simulink model "primera_parte"  (R2023a)
settings: Solver=VariableStepAuto  StartTime=0.0  StopTime=3  RelTol=1e-3
values from neighbouring files (symbols this model uses):
  A = [a11 a21 a12 a22]    [calc_A.m]    (also in modelo.m = [a11 a12)
  Ad = [-1/t_beta 0 ... (first row only)    [calc_KMax.m]    (also in calc_Kmin.m; modelo.m)
  B = [b11 b21 b12 b22]    [calc_B.m]    (also in calc_inv_B.m = [b11 b12; b21 b22]; modelo.m = [b11 b12)
  C = [1 0 ... (first row only)    [modelo.m]
  D = [0 0;0 0]    [modelo.m]
  E = [e1 e2]    [calc_E.m]    (also in modelo.m = [e1)
  Ed = [k_beta/t_beta ... (first row only)    [calc_KMax.m]    (also in calc_Kmin.m; modelo.m)
  k = double(Y)*inv(double(P))    [calc_KMax.m]    (also in calc_Kmin.m; modelo.m = H_inf_robust(A1,A2,B11,B12,B21,B22,C1,D12,D11))
  x0 = [0, 0]    [modelo.m]
undefined symbols (not defined in the file or in its folder): sigbuilder_block
settings Model: Creator=Ferna  LastModifiedBy=Ferna
settings DebuggingCC: UnconnectedInputMsg=warning  UnconnectedOutputMsg=warning  UnconnectedLineMsg=warning
settings ModelReferenceCC: EnableRefExpFcnMdlSchedulingChecks=on
settings RTWCC: DLArmComputeVersion=19.05

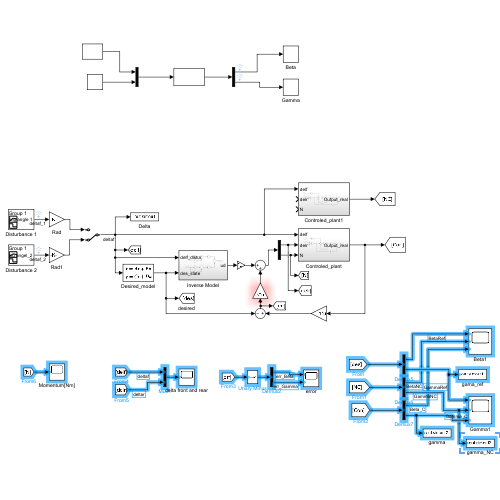
[thumbnail: Simulink's stored preview of the top-level diagram]
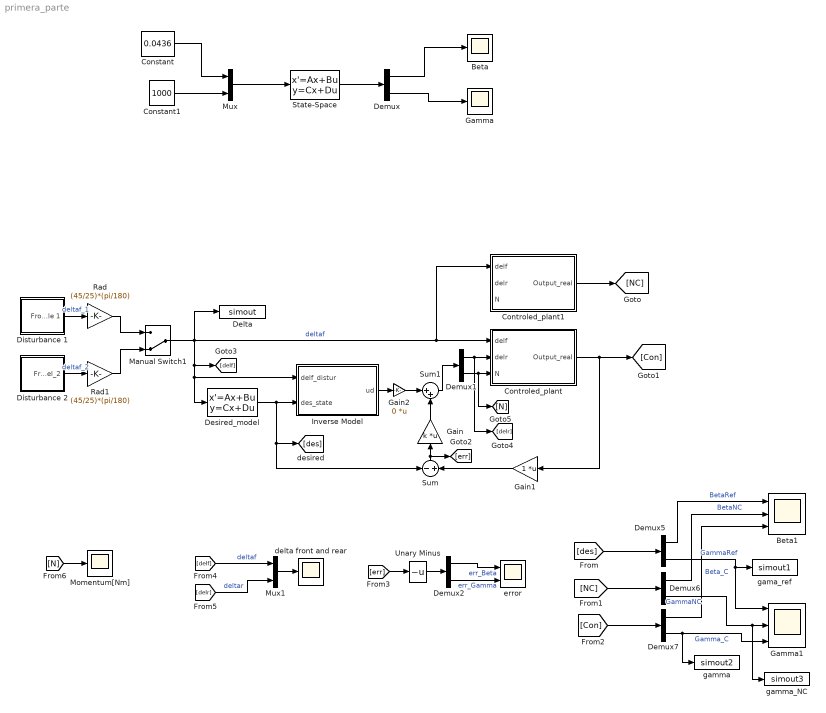
== system primera_parte ==
  Beta : Scope
  Beta1 : Scope  NumInputPorts=3
  Constant : Constant  Value=0.0436
  Constant1 : Constant  Value=1000
  Controled_plant : Subsystem
  Controled_plant1 : Subsystem
  Delta : ToWorkspace  VariableName=simout  SaveFormat=Timeseries  SampleTime=-1
  Demux{,1..2,5..7} (6 alike) : Demux  Outputs=2
  Desired_model : StateSpace  A=Ad  B=Ed  C=[1,0;0,1]  D=zeros(2,1)  InitialCondition=0
  Disturbance 1 : Subsystem  Tag=STV Subsys  LoadFcn=sigbuilder_block('load');  StartFcn=sigbuilder_block('start');  StopFcn=sigbuilder_block('stop');  ClipboardFcn=sigbuilder_block('clipboard');  mask(Sigbuilder block){tuvar=[0:10]}
      mask help: Simulink:masks:SigbuilderBlock_MD
      mask init:
      | if ~strcmp(get_param(bdroot(gcbh),'SimulationStatus'),'stopped') tuvar = sigbuilder_block('maskInit'); end
      settings: CopyFcn=sigbuilder_block('copy');  DeleteFcn=sigbuilder_block('delete');  ModelCloseFcn=sigbuilder_block('modelClose');  PreSaveFcn=sigbuilder_block('preSave');  PauseFcn=sigbuilder_block('pause');  ContinueFcn=sigbuilder_block('continue');  NameChangeFcn=sigbuilder_block('namechange');  OpenFcn=sigbuilder_block('open',[265.8 141.6 550.8 400.2 ]);  CloseFcn=sigbuilder_block('close');
      mask Display: plot(0, 0, 100, 100,[2, 2, 32, 32, 2], [68, 8, 8, 68, 68],[32, 2], [38, 38], [32, 19, 2],[53, 60, 44], [32, 17, 17, 2],[16, 16, 31, 31]);txt = getActiveGroup(gcbh);text(2, 100, txt,'verticalAlignment', 'top');
  Disturbance 2 : Subsystem  Tag=STV Subsys  LoadFcn=sigbuilder_block('load');  StartFcn=sigbuilder_block('start');  StopFcn=sigbuilder_block('stop');  ClipboardFcn=sigbuilder_block('clipboard');  mask(Sigbuilder block){tuvar=[0:10]}
      mask help: Simulink:masks:SigbuilderBlock_MD
      mask init:
      | if ~strcmp(get_param(bdroot(gcbh),'SimulationStatus'),'stopped') tuvar = sigbuilder_block('maskInit'); end
      settings: CopyFcn=sigbuilder_block('copy');  DeleteFcn=sigbuilder_block('delete');  ModelCloseFcn=sigbuilder_block('modelClose');  PreSaveFcn=sigbuilder_block('preSave');  PauseFcn=sigbuilder_block('pause');  ContinueFcn=sigbuilder_block('continue');  NameChangeFcn=sigbuilder_block('namechange');  OpenFcn=sigbuilder_block('open',[265.8 141.6 550.8 400.2 ]);  CloseFcn=sigbuilder_block('close');
      mask Display: plot(0, 0, 100, 100,[2, 2, 32, 32, 2], [68, 8, 8, 68, 68],[32, 2], [38, 38], [32, 19, 2],[53, 60, 44], [32, 17, 17, 2],[16, 16, 31, 31]);txt = getActiveGroup(gcbh);text(2, 100, txt,'verticalAlignment', 'top');
  Gain : Gain  Gain=k  Multiplication=Matrix(K*u)
  Gain1 : Gain  Multiplication=Matrix(K*u)
  Gain2 : Gain  Gain=0  Multiplication=Matrix(K*u)
  Gamma : Scope
  Gamma1 : Scope  NumInputPorts=3
  Inverse Model : Subsystem
  Manual Switch1 : ManualSwitch  CurrentSetting=0
  Momentum[Nm] : Scope
  Mux : Mux  Inputs=2
  Mux1 : Mux  Inputs=2
  Rad : Gain  Gain=(45/25)*(pi/180)
  Rad1 : Gain  Gain=(45/25)*(pi/180)
  State-Space : StateSpace  A=A  B=B  C=C  D=D  InitialCondition=x0
  Sum : Sum  Inputs=-|+
  Sum1 : Sum  Inputs=|++
  Unary Minus : UnaryMinus
  delta front and rear : Scope
  error : Scope  NumInputPorts=2
  gama_ref : ToWorkspace  VariableName=simout1  SaveFormat=Timeseries  SampleTime=-1
  gamma : ToWorkspace  VariableName=simout2  SaveFormat=Timeseries  SampleTime=-1
  gamma_NC : ToWorkspace  VariableName=simout3  SaveFormat=Timeseries  SampleTime=-1
  wires:
  Mux/1 -> State-Space/1
  Constant/1 -> Mux/1
  Constant1/1 -> Mux/2
  State-Space/1 -> Demux/1
  Demux/1 -> Beta/1
  Demux/2 -> Gamma/1
  Disturbance 1/1(Front sterring angle 1) -> Rad/1  "deltaf_1"
  Disturbance 2/1(Front steering angel_2) -> Rad1/1  "deltaf_2"
  Rad/1 -> Manual Switch1/1
  Rad1/1 -> Manual Switch1/2
  Manual Switch1/1 -> Delta/1, Controled_plant1/1(delf), Controled_plant/1(delf), [delf], Inverse Model/1(delf_distur), Desired_model/1  "deltaf"
  Desired_model/1 -> [des], Sum/1, Inverse Model/2(des_state)
  Controled_plant/1(Output_real) -> Gain1/1, [Con]
  Sum/1 -> [err], Gain/1
  Gain/1 -> Sum1/2
  Demux1/1 -> [delr], Controled_plant/2(delr)
  Demux1/2 -> [N], Controled_plant/3(N)
  Sum1/1 -> Demux1/1
  Controled_plant1/1(Output_real) -> [NC]
  Gain1/1 -> Sum/2
  [des] -> Demux5/1
  [NC] -> Demux6/1
  Demux5/1 -> Beta1/1  "BetaRef"
  Demux6/1 -> Beta1/2  "BetaNC"
  Demux7/1 -> Beta1/3  "Beta_C"
  [Con] -> Demux7/1
  Demux5/2 -> gama_ref/1, Gamma1/1  "GammaRef"
  Demux6/2 -> gamma_NC/1, Gamma1/2  "GammaNC"
  Demux7/2 -> gamma/1, Gamma1/3  "Gamma_C"
  Inverse Model/1(ud) -> Gain2/1
  Gain2/1 -> Sum1/1
  [err] -> Unary Minus/1
  Unary Minus/1 -> Demux2/1
  Demux2/1 -> error/1  "err_Beta"
  Demux2/2 -> error/2  "err_Gamma"
  [delf] -> Mux1/1  "deltaf"
  [delr] -> Mux1/2  "deltar"
  Mux1/1 -> delta front and rear/1
  [N] -> Momentum[Nm]/1

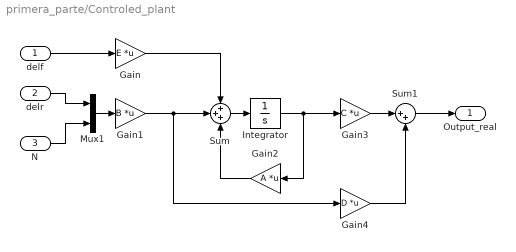
== system primera_parte/Controled_plant ==
  delf : Inport
  delr : Inport  Port=2
  N : Inport  Port=3
  Gain : Gain  Gain=E  Multiplication=Matrix(K*u)
  Gain1 : Gain  Gain=B  Multiplication=Matrix(K*u)
  Gain2 : Gain  Gain=A  Multiplication=Matrix(K*u)
  Gain3 : Gain  Gain=C  Multiplication=Matrix(K*u)
  Gain4 : Gain  Gain=D  Multiplication=Matrix(K*u)
  Integrator : Integrator  InitialCondition=x0
  Mux1 : Mux  Inputs=2
  Sum : Sum  Inputs=+++
  Sum1 : Sum  Inputs=|++
  Output_real : Outport
  wires:
  Gain1/1 -> Gain4/1, Sum/2
  Gain4/1 -> Sum1/2
  delr/1 -> Mux1/1
  delf/1 -> Gain/1
  Integrator/1 -> Gain3/1, Gain2/1
  Gain/1 -> Sum/1
  Sum1/1 -> Output_real/1
  Gain3/1 -> Sum1/1
  N/1 -> Mux1/2
  Mux1/1 -> Gain1/1
  Sum/1 -> Integrator/1
  Gain2/1 -> Sum/3

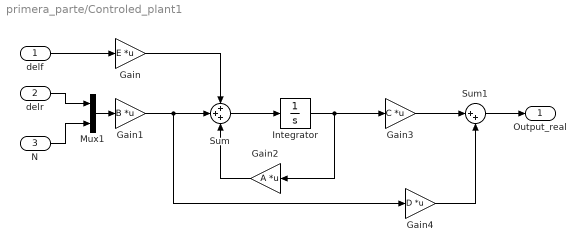
== system primera_parte/Controled_plant1 ==
  delf : Inport
  delr : Inport  Port=2
  N : Inport  Port=3
  Gain : Gain  Gain=E  Multiplication=Matrix(K*u)
  Gain1 : Gain  Gain=B  Multiplication=Matrix(K*u)
  Gain2 : Gain  Gain=A  Multiplication=Matrix(K*u)
  Gain3 : Gain  Gain=C  Multiplication=Matrix(K*u)
  Gain4 : Gain  Gain=D  Multiplication=Matrix(K*u)
  Integrator : Integrator  InitialCondition=x0
  Mux1 : Mux  Inputs=2
  Sum : Sum  Inputs=+++
  Sum1 : Sum  Inputs=|++
  Output_real : Outport
  wires:
  Gain2/1 -> Sum/3
  Sum/1 -> Integrator/1
  Mux1/1 -> Gain1/1
  N/1 -> Mux1/2
  Gain3/1 -> Sum1/1
  Sum1/1 -> Output_real/1
  Gain/1 -> Sum/1
  Integrator/1 -> Gain2/1, Gain3/1
  delf/1 -> Gain/1
  delr/1 -> Mux1/1
  Gain4/1 -> Sum1/2
  Gain1/1 -> Sum/2, Gain4/1

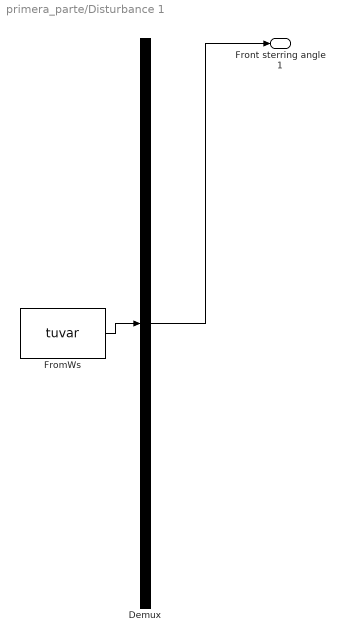
== system primera_parte/Disturbance 1 ==
  Demux : Demux  Tag=STV Demux  Outputs=1
      settings: DisplayOption=none
  FromWs : FromWorkspace  Tag=STV FromWs  VariableName=tuvar
      SigBuilderData=|
      | common.afterFinalStr = 'Extrapolate'
      | common.sampleTime = 0
      | dataSet.timeRange = [0 3]
      | dataSet.name = 'Group 1'
      | sbobj.Groups.Name = 'Group 1'
      | sbobj.Groups.Signals.Name = 'Front sterring angle 1'
      | sbobj.Groups.Signals.XData = [0 0.5 0.66 0.88 1.01 2.5 3]
      | sbobj.Groups.Signals.YData = [-0.01 0 0.2 0.8 1 1 1]
      | sbobj.Groups.TimeRange = [0 3]
  Front sterring angle 1 : Outport  Tag=STV Outport
  wires:
  FromWs/1 -> Demux/1
  Demux/1 -> Front sterring angle 1/1

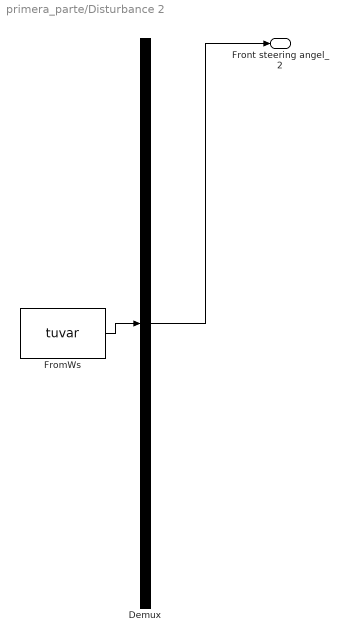
== system primera_parte/Disturbance 2 ==
  Demux : Demux  Tag=STV Demux  Outputs=1
      settings: DisplayOption=none
  FromWs : FromWorkspace  Tag=STV FromWs  VariableName=tuvar
      SigBuilderData=|
      | common.afterFinalStr = 'Extrapolate'
      | common.sampleTime = 0
      | dataSet.timeRange = [0 3]
      | dataSet.name = 'Group 1'
      | sbobj.Groups.Name = 'Group 1'
      | sbobj.Groups.Signals.Name = 'Front steering angel_2'
      | sbobj.Groups.Signals.XData = [0 0.187490625469 0.374981250937 0.562471876406 0.749962501875 0.937453127344 1.12494375281 1.31243437828 1.49992500375 1.68741562922 1.87490625469 2.06239688016 2.24988750562 2.43737813109 2.62486875656 2.81235938203 2.9998500075 3]
      | sbobj.Groups.Signals.YData = [0 0.565685424949 0.8 0.565685424949 9.79717439318e-17 -0.565685424949 -0.8 -0.565685424949 0 0 0 0 0 0 0 0 0 0]
      | sbobj.Groups.TimeRange = [0 3]
  Front steering angel_2 : Outport  Tag=STV Outport
  wires:
  Demux/1 -> Front steering angel_2/1
  FromWs/1 -> Demux/1

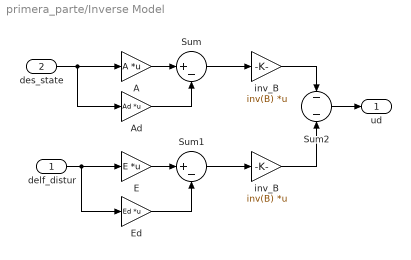
== system primera_parte/Inverse Model ==
  delf_distur : Inport
  des_state : Inport  Port=2
  A : Gain  Gain=A  Multiplication=Matrix(K*u)
  Ad : Gain  Gain=Ad  Multiplication=Matrix(K*u)
  E : Gain  Gain=E  Multiplication=Matrix(K*u)
  Ed : Gain  Gain=Ed  Multiplication=Matrix(K*u)
  Sum : Sum  Inputs=|+-
  Sum1 : Sum  Inputs=|+-
  Sum2 : Sum  Inputs=-|-
  inv_B : Gain  Gain=inv(B)  Multiplication=Matrix(K*u)
  "inv_B " : Gain  Gain=inv(B)  Multiplication=Matrix(K*u)
  ud : Outport
  wires:
  E/1 -> Sum1/1
  Ad/1 -> Sum/2
  inv_B/1 -> Sum2/1
  delf_distur/1 -> Ed/1, E/1
  "inv_B "/1 -> Sum2/2
  Sum/1 -> inv_B/1
  A/1 -> Sum/1
  des_state/1 -> Ad/1, A/1
  Sum1/1 -> "inv_B "/1
  Sum2/1 -> ud/1
  Ed/1 -> Sum1/2
